simulink model "AMgeneration"  (R2013a)
settings: Solver=VariableStepDiscrete  SolverMode=SingleTasking  StartTime=0.0  StopTime=10  RelTol=1e-3
libraries: powerlib_meascontrol x1
settings Model: Creator=student  LastModifiedBy=senthilkumar
settings DataIOCC: SaveOutput=off  SaveTime=off
settings OptimizationCC: BooleanDataType=off  InlineParams=on  LocalBlockOutputs=off
settings DebuggingCC: AlgebraicLoopMsg=error  SingleTaskRateTransMsg=error

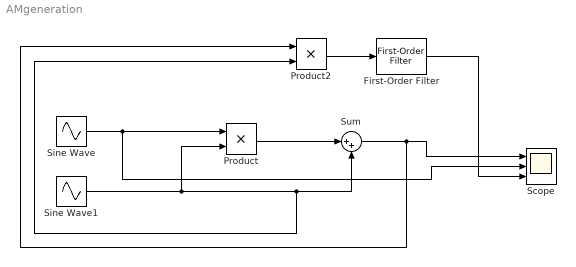
== system AMgeneration ==
  First-Order Filter : powerlib_meascontrol/Filters/First-Order Filter  FilterType=Lowpass  Tc=10e-3  Ts=0.00005  Initialize=on  Vac_Init=[0, 0, 60]  Vdc_Init=0  PlotResponse=off  FreqRange="[0,  200,  1]"
  Product : Product
  Product2 : Product
  Scope : Scope  NumInputPorts=3
      settings: YMin=-5~-10~-5  YMax=5~10~5
  Sine Wave : Sin  Amplitude=.5  Frequency=50  SampleTime=0.00005
  Sine Wave1 : Sin  Frequency=10000  SampleTime=0.00005
  Sum : Sum  Inputs=|++
  wires:
  Sine Wave/1 -> Scope/2, Product/1
  Sine Wave1/1 -> Product2/2, Sum/2, Product/2
  Product/1 -> Sum/1
  Sum/1 -> Product2/1, Scope/1
  Product2/1 -> First-Order Filter/1
  First-Order Filter/1 -> Scope/3
